simulink model "DD20220405"  (R2021a)
settings: Solver=VariableStepAuto  StartTime=0.0  StopTime=200  RelTol=1e-3
undefined symbols (not defined in the file): B, K1, K2, M1, M2
settings Model: Creator=jaewan  LastModifiedBy=jaewan

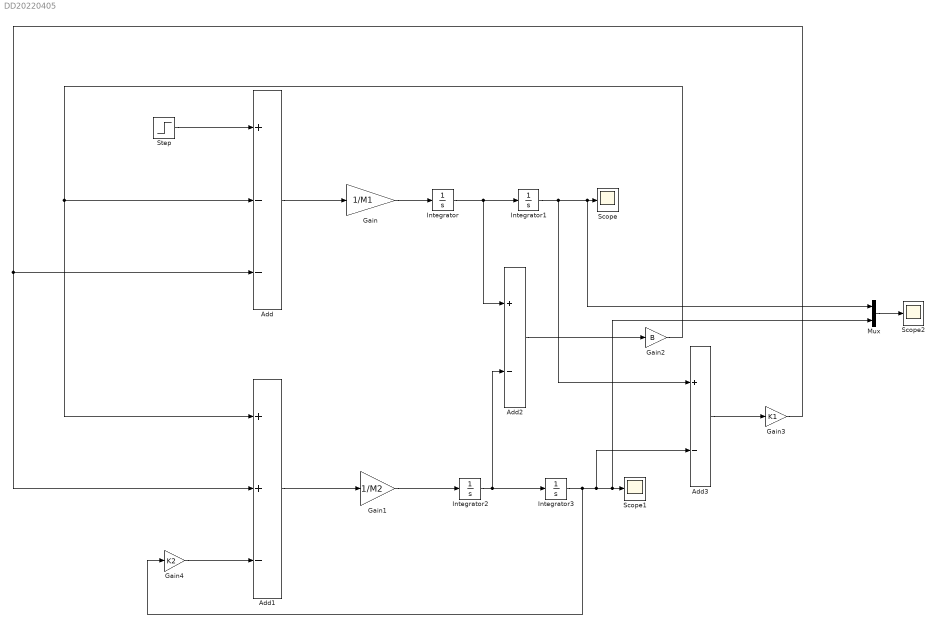
== system DD20220405 ==
  Add : Sum  Inputs=+--
  Add1 : Sum  Inputs=++-
  Add2 : Sum  Inputs=+-
  Add3 : Sum  Inputs=+-
  Gain : Gain  Gain=1/M1
  Gain1 : Gain  Gain=1/M2
  Gain2 : Gain  Gain=B
  Gain3 : Gain  Gain=K1
  Gain4 : Gain  Gain=K2
  Integrator{,1..3} (4 alike) : Integrator
  Mux : Mux  Inputs=2
  Scope : Scope
  Scope1 : Scope
  Scope2 : Scope
  Step : Step  After=8  SampleTime=0
  wires:
  Add/1 -> Gain/1
  Gain/1 -> Integrator/1
  Integrator/1 -> Add2/1, Integrator1/1
  Integrator1/1 -> Mux/1, Scope/1, Add3/1
  Integrator3/1 -> Gain4/1, Add3/2, Mux/2, Scope1/1
  Integrator2/1 -> Integrator3/1, Add2/2
  Gain1/1 -> Integrator2/1
  Add1/1 -> Gain1/1
  Add2/1 -> Gain2/1
  Gain2/1 -> Add1/1, Add/2
  Step/1 -> Add/1
  Add3/1 -> Gain3/1
  Gain3/1 -> Add/3, Add1/2
  Gain4/1 -> Add1/3
  Mux/1 -> Scope2/1
